simulink model "generic_AEL"  (R2024b)
settings: Solver=VariableStepAuto  StartTime=0.0  StopTime=30  RelTol=1e-3
libraries: spsSeriesRLCBranchLib x4, spsCurrentMeasurementLib x3, spsVariableResistorLib x2, spsVoltageMeasurementLib x2, spsDCVoltageSourceLib x1, spsControlledCurrentSourceLib x1, simulink x1, sps_lib x1
settings Model: Creator=luxali  LastModifiedBy=luxali
settings RTWCC: GPUComputeCapability=3.5

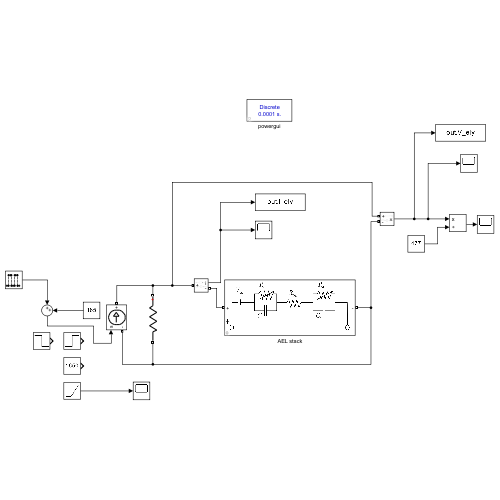
[thumbnail: Simulink's stored preview of the top-level diagram]
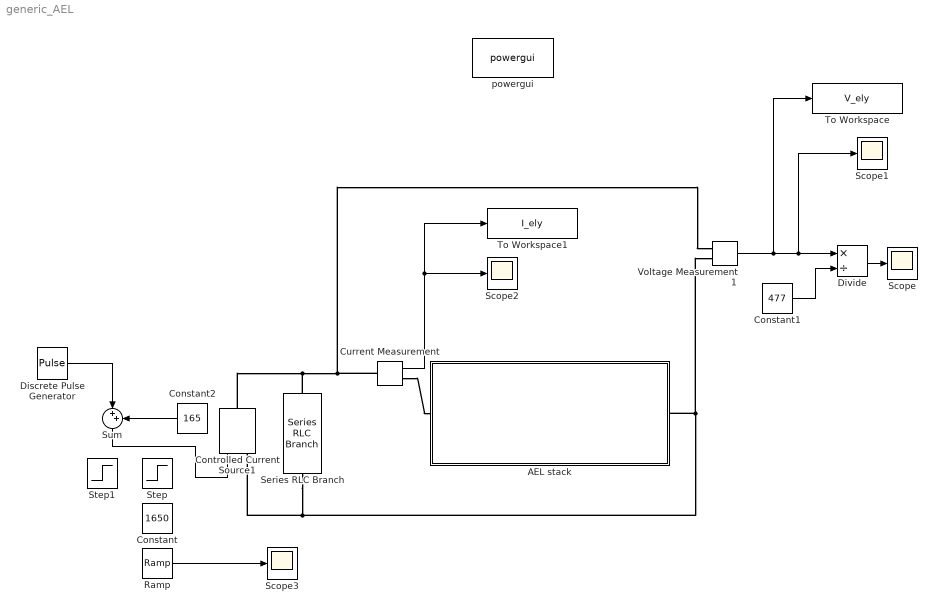
== system generic_AEL ==
  AEL stack : Subsystem  mask{I0_a=1650, I0_c=1650, V0_a_cell=0.25, V0_c_cell=0.25, A_cell=10000, N_cell=477, P_min_share=10, P_max_share=100, i_nom=0.165, ResultPIV=|, R_cell_ohm=0.89, Ca=1, Cc=100, a=0.04, c=0.12, i0=1.2e-4, V_rev=1.26}
      mask ResultPIV=|
      | Nominal power in kW: 1502.46
      | Operating power range in kW: 150.25 - 1502.46
      |
      | Nominal voltage in V: 910.58
      | Nominal current in A: 1650.00
      mask prompts: I0_a "Initial resistor current at anode in A"; I0_c "Initial resistor current at cathode in A"; V0_a_cell "Initial capacitor anode cell voltage in V"; V0_c_cell "Initial capacitor cathode cell voltage in V"; A_cell "Cell active area A_cell in cm^2"; N_cell "Number of cells N_cell"; P_min_share "Minimum power in %"; P_max_share "Maximum power in %"; i_nom "Nominal current desnity in A/cm^2"; R_cell_ohm "Ohmic cell resistance in Ohm/cm^2"; Ca "Anode cell capacity in mF/cm^2"; Cc "Cathode cell capacity in mF/cm^2"; a "Anode tafel slope in V/dec"; c "Cathode tafel slope in V/dec"; i0 "Exchange current density in A/cm^2"; V_rev "Reversible cell voltage in V"
      mask DialogControl DescTextVar Prompt: Alkaline electrolyzer
      mask DialogControl Control4 Prompt: The generic alkaline electrolyzer model is based on an equivalent circuit model structure. The cathode and anode resistant are dependent on the current, wherefore initial conditions are required. Initial voltage values are needed for the constant capacitors. When connecting a current source to the electrolyzer model, the direction needs to be considered as marked. The calculated operation range does not limit the current input and is for information display only.
      mask DialogControl Container5 Prompt: References
      mask DialogControl Control5 Prompt: For more information About the model structure, see the AGISTIN Deliverable D3.2. The default parameters are taken from Sanchez-Ruiz and de Groot (https://doi.org/10.1016/j.ijhydene.2024.11.372).
      mask DialogControl Control3 Prompt: Copyright © by Fraunhofer IWES
      mask DialogControl PIV_calc Prompt: Get: power / voltage / current
      mask DialogControl PIV_calc Tooltip: Press button for calculation
      mask DialogControl Container3 Prompt: Model parameters
      mask DialogControl Container4 Prompt: Initial conditions
      mask Display: image('Mask_pic.png');
  Constant : Constant  Value=1650
  Constant1 : Constant  Value=477
  Constant2 : Constant  Value=165
  Controlled Current Source1 : spsControlledCurrentSourceLib/Controlled Current Source  Initialize=on  Source_Type=DC  Amplitude=0  Phase=0  Frequency=0  Measurements=None
  Current Measurement : spsCurrentMeasurementLib/Current Measurement  PhasorSimulation=off  OutputType=Complex  PSBequivalent=0
  Discrete Pulse Generator : DiscretePulseGenerator  Amplitude=1650-165  Period=10  PulseWidth=5
  Divide : Product  Inputs=*/
  Ramp : simulink/Sources/Ramp  slope=165  start=0  InitialOutput=16.5
  Scope{,1..3} (4 alike) : Scope
  Series RLC Branch : spsSeriesRLCBranchLib/Series RLC Branch  LConnTagsString=__new0  RConnTagsString=__new0  BranchType=R  Resistance=1e6  Inductance=1e-3  SetiL0=off  InitialCurrent=0  Capacitance=1e-6  Setx0=off  InitialVoltage=0  Measurements=None
  Step : Step  Time=10  Before=165  After=1650  SampleTime=0
  Step1 : Step  Time=10  Before=1650  After=165  SampleTime=0
  Sum : Sum  Inputs=|++
  To Workspace : ToWorkspace  VariableName=V_ely  SaveFormat=Timeseries  SampleTime=-1
  To Workspace1 : ToWorkspace  VariableName=I_ely  SaveFormat=Timeseries  SampleTime=-1
  Voltage Measurement1 : spsVoltageMeasurementLib/Voltage Measurement  PhasorSimulation=off  OutputType=Complex  PSBequivalent=0
  powergui : sps_lib/powergui  Priority=1  SimulationMode=Discrete  SampleTime=1e-4  frequency=60  Iterations=50  frequencyindice=0  Pbase=100e6  ErrMax=1e-4  UnitsV=kV  UnitsW=MW  buscounter=0  FunctionMessages=off  echomessages=off  EnableUseOfTLC=off  CurrentSourceSwitches=off  DisableSnubberDevices=off  DisableRonSwitches=off  DisableVfSwitches=off  DisplayEquations=off  AutomaticDiscreteSolvers=off  SolverType=Tustin/Backward Euler (TBE)  Interpol=off  ExternalGateDelay=off  methode=off  Ts=100  x0status=blocks  SPID=on  SwTol=0  HookPort=off  NonlinearTolerance=1e-4  nMaxIteration=100  ContinueOnMaxIteration=off  RestoreLinks=warning  ResistiveCurrentMeasurement=off  Frange=[0:2:500]  Ylog=off  Xlog=on  ShowGrid=off  save=off  variable=ZData  structure=0  ZoomFFT=off  StartTime=0.0  cycles=1  DisplayStyle=1  fundamental=60  FreqAxis=off  MaxFrequency=1000  frequencyindicesteady=1  RmsSteady=1  display=off
  wires:
  Voltage Measurement1/1 -> To Workspace/1, Scope1/1, Divide/1
  Current Measurement/1 -> To Workspace1/1, Scope2/1
  Constant1/1 -> Divide/2
  Divide/1 -> Scope/1
  Discrete Pulse Generator/1 -> Sum/1
  Constant2/1 -> Sum/2
  Sum/1 -> Controlled Current Source1/1
  Ramp/1 -> Scope3/1
  connections:
  Series RLC Branch/RConn1 -- Voltage Measurement1/LConn2 -- AEL stack/RConn1 -- Controlled Current Source1/LConn1
  Controlled Current Source1/RConn1 -- Series RLC Branch/LConn1 -- Voltage Measurement1/LConn1 -- Current Measurement/LConn1
  Current Measurement/RConn1 -- AEL stack/LConn1

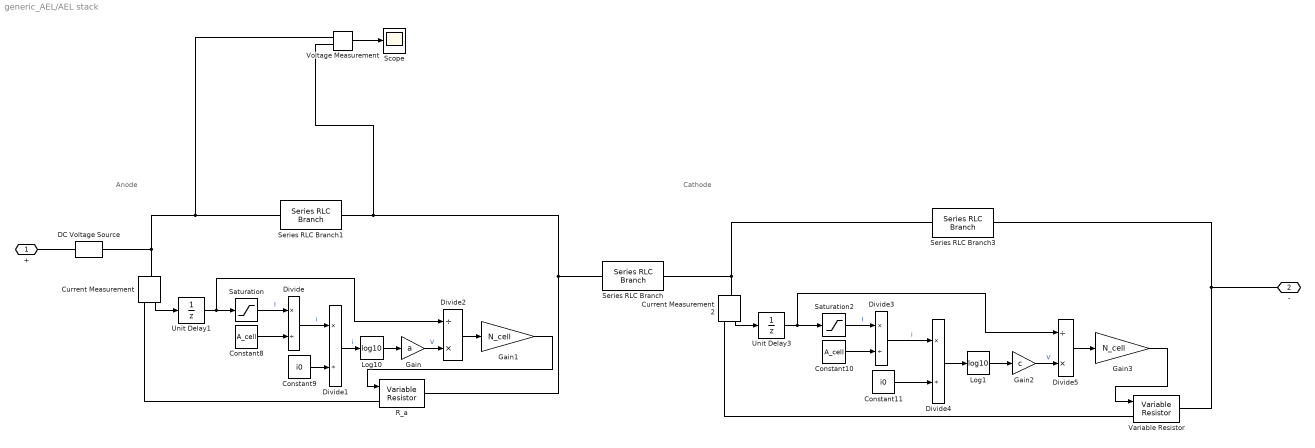
== system generic_AEL/AEL stack ==
  note: Cathode
  note: Anode
  Constant10 : Constant  Value=A_cell
  Constant11 : Constant  Value=i0
  Constant8 : Constant  Value=A_cell
  Constant9 : Constant  Value=i0
  Current Measurement : spsCurrentMeasurementLib/Current Measurement  PhasorSimulation=off  OutputType=Complex  PSBequivalent=0
  Current Measurement2 : spsCurrentMeasurementLib/Current Measurement  PhasorSimulation=off  OutputType=Complex  PSBequivalent=0
  DC Voltage Source : spsDCVoltageSourceLib/DC Voltage Source  Amplitude=V_rev*N_cell  Measurements=None
  Divide{,1,3..4} (4 alike) : Product  Inputs=*/
  Divide2 : Product  Inputs=/*
  Divide5 : Product  Inputs=/*
  Gain : Gain  Gain=a
  Gain1 : Gain  Gain=N_cell
  Gain2 : Gain  Gain=c
  Gain3 : Gain  Gain=N_cell
  Log1 : Math  Operator=log10
  Log10 : Math  Operator=log10
  R_a : spsVariableResistorLib/Variable Resistor  Rabsmin=1e-3
      settings: LibrarySourceBlock=sps_lib/Passives/Variable Resistor
  Saturation : Saturate  UpperLimit=inf  LowerLimit=1e-3
  Saturation2 : Saturate  UpperLimit=inf  LowerLimit=1e-3
  Scope : Scope
  Series RLC Branch : spsSeriesRLCBranchLib/Series RLC Branch  LConnTagsString=__new0  RConnTagsString=__new0  BranchType=R  Resistance=R_cell_ohm/A_cell*N_cell  Inductance=1e-3  SetiL0=off  InitialCurrent=0  Capacitance=1e-6  Setx0=off  InitialVoltage=0  Measurements=None
  Series RLC Branch1 : spsSeriesRLCBranchLib/Series RLC Branch  LConnTagsString=__new0  RConnTagsString=__new0  BranchType=C  Resistance=1  Inductance=1e-3  SetiL0=off  InitialCurrent=0  Capacitance=Ca*A_cell *1e-3/N_cell  Setx0=on  InitialVoltage=V0_a_cell*N_cell  Measurements=None
  Series RLC Branch3 : spsSeriesRLCBranchLib/Series RLC Branch  LConnTagsString=__new0  RConnTagsString=__new0  BranchType=C  Resistance=1  Inductance=1e-3  SetiL0=off  InitialCurrent=0  Capacitance=Cc*A_cell *1e-3/N_cell  Setx0=on  InitialVoltage=V0_a_cell*N_cell  Measurements=None
  Unit Delay1 : UnitDelay  InitialCondition=I0_a  SampleTime=-1  HasFrameUpgradeWarning=on
  Unit Delay3 : UnitDelay  InitialCondition=I0_c  SampleTime=-1  HasFrameUpgradeWarning=on
  Variable Resistor : spsVariableResistorLib/Variable Resistor  Rabsmin=1e-3
      settings: LibrarySourceBlock=sps_lib/Passives/Variable Resistor
  Voltage Measurement : spsVoltageMeasurementLib/Voltage Measurement  PhasorSimulation=off  OutputType=Complex  PSBequivalent=0
  + : PMIOPort  Side=Left
  - : PMIOPort  Port=2  Side=Right
  wires:
  Saturation/1 -> Divide/1  "I"
  Constant8/1 -> Divide/2
  Gain/1 -> Divide2/2  "V"
  Gain1/1 -> R_a/1
  Divide2/1 -> Gain1/1
  Log10/1 -> Gain/1
  Current Measurement/1 -> Unit Delay1/1
  Current Measurement2/1 -> Unit Delay3/1
  Saturation2/1 -> Divide3/1  "I"
  Gain3/1 -> Variable Resistor/1
  Constant10/1 -> Divide3/2
  Divide5/1 -> Gain3/1
  Gain2/1 -> Divide5/2  "V"
  Divide4/1 -> Log1/1
  Log1/1 -> Gain2/1
  Constant11/1 -> Divide4/2
  Divide3/1 -> Divide4/1  "i"
  Divide/1 -> Divide1/1  "i"
  Constant9/1 -> Divide1/2
  Divide1/1 -> Log10/1  "i"
  Unit Delay1/1 -> Saturation/1, Divide2/1
  Unit Delay3/1 -> Divide5/1, Saturation2/1
  Voltage Measurement/1 -> Scope/1
  connections:
  R_a/RConn1 -- Voltage Measurement/LConn2 -- Series RLC Branch1/RConn1 -- Series RLC Branch/LConn1
  +/RConn1 -- DC Voltage Source/RConn1
  Current Measurement/RConn1 -- R_a/LConn1
  Series RLC Branch/RConn1 -- Current Measurement2/LConn1 -- Series RLC Branch3/LConn1
  Current Measurement2/RConn1 -- Variable Resistor/LConn1
  -/RConn1 -- Variable Resistor/RConn1 -- Series RLC Branch3/RConn1
  DC Voltage Source/LConn1 -- Current Measurement/LConn1 -- Voltage Measurement/LConn1 -- Series RLC Branch1/LConn1
